simulink model "momentum_dumping"  (R2023b)
settings: Solver=VariableStepAuto  StartTime=0.0  StopTime=30  FixedStep=0.  RelTol=2.8421709430404007E-14
model workspace (MAT data in the model file):
  x0 = 0
values from neighbouring files (symbols this model uses):
  A_BP = A_PB'    [mass_properties.m]
  A_PB = [e1_B'; e2_B'; e3_B']    [mass_properties.m]
  dt_delay = 0.01    [main_momentum.m]
  hwdotmax = 0.004    [main_momentum.m]
  hwmax = 0.015    [main_momentum.m]
  hwstar_B = [0;0;0]    [main_momentum.m]
  J_C_B = Js_C_B + Jd_C_B    [mass_properties.m]
  K = 1/bode(Co*CLTF1*Go,w_crossover_o)    [main_momentum.m]
  Kd = diag([Kd1; Kd2; Kd3])    [main_momentum.m]
  Km = 1/bode(Gm, 2*pi*0.001)    [main_momentum.m]
  Kp = 1/bode(CLTF1/s, 2*pi*0.92244)    [main_momentum.m]
  md = 0.05290847    [mass_properties.m]
  Mmax = 0.17    [main_momentum.m]
  ms = 3.21000120    (= 3.2100012)    [mass_properties.m]
  p = 100*2*pi    (= 628.318530718)    [main_momentum.m]
  q_PB = A2q(A_PB)    [mass_properties.m]
  qstar_BI = e2q(e,150*pi/180)    [main_momentum.m]
  rcb_B = ((ms * rsb_B) + (md * rdb_B)) / (ms + md)    [mass_properties.m]
  rlb_B = [0.16364; -0.03142; -0.02136]    [mass_properties.m]
  s = tf('s')    [main_momentum.m]
  safety = 0.5    [main_momentum.m]
  tau = 1/(100*2*pi)    (= 0.00159154943092)    [main_momentum.m]
  wn = 2*pi*10    (= 62.8318530718)    [main_momentum.m]
  z = 0.006*2*pi    (= 0.0376991118431)    [main_momentum.m]
  zeta = sqrt(2)/2    [main_momentum.m]
undefined symbols (not defined in the file or in its folder): input, input_dis, q0_BI, X, Y, Z
libraries: sm_lib x10, nesl_utility x4, matrix_library x1
settings Model: Creator=bbingham  LastModifiedBy=alanb
settings SolverCC: AlgebraicLoopSolver=TrustRegion
settings DataIOCC: SaveOutput=off  SignalLogging=off  DSMLogging=off  ReturnWorkspaceOutputs=off
settings DebuggingCC: UnconnectedInputMsg=warning  UnconnectedOutputMsg=warning  UnconnectedLineMsg=warning  ArithmeticOperatorsInVariantConditions=warning
settings ModelReferenceCC: EnableRefExpFcnMdlSchedulingChecks=on
settings SFSimCC: SimUseLocalCustomCode=off  CustomCodeUndefinedFunction=UseInterfaceOnly
settings RTWCC: Description=Simulink Desktop Real-Time  SystemTargetFile=sldrt.tlc  TemplateMakefile=sldrt.tmf  RTWUseLocalCustomCode=off  RTWCompilerOptimization=on
settings CodeAppCC: MaxIdLength=95  StateflowObjectComments=on
settings SimulinkDesktopRealTimeCC: TargetPreCompLibLocation=C:\Program Files\MATLAB\R2020a\toolbox\sldrt\lib\win64
settings SimscapeCC: SimscapeNormalizeSystem=off

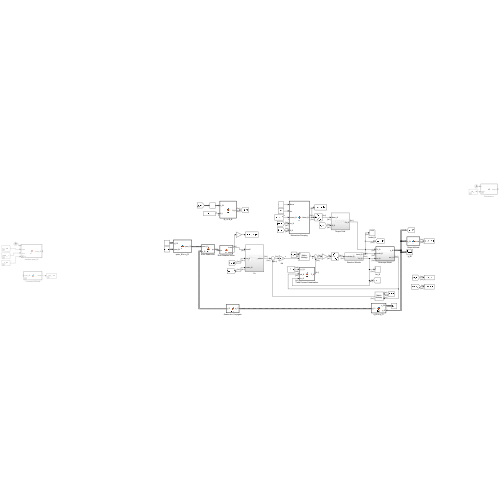
[thumbnail: Simulink's stored preview of the top-level diagram]
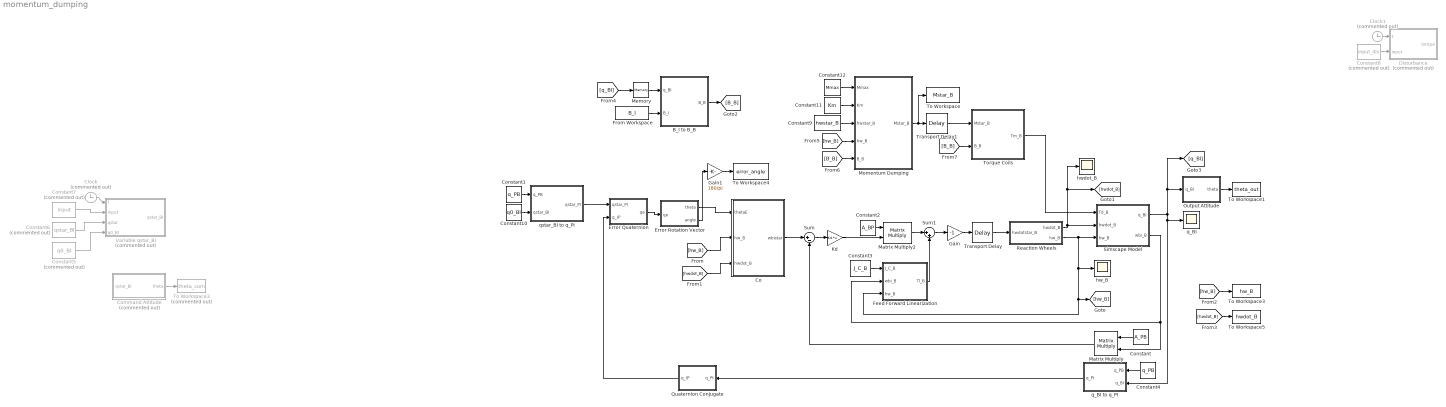
== system momentum_dumping ==
  B_I to B_B : MATLAB Function  TreatAsAtomicUnit=on
  Clock : Clock  Commented=on
  Clock1 : Clock  Commented=on
  Co : Subsystem
  Command Attitude : MATLAB Function  Commented=on  TreatAsAtomicUnit=on
  Constant : Constant  Value=A_PB
  Constant1 : Constant  Value=q_PB  OutDataTypeStr=Bus: qBus
  Constant10 : Constant  Value=q0_BI  OutDataTypeStr=Bus: qBus
  Constant11 : Constant  Value=Km
  Constant12 : Constant  Value=Mmax
  Constant2 : Constant  Value=A_BP
  Constant3 : Constant  Value=J_C_B
  Constant4 : Constant  Value=q_PB  OutDataTypeStr=Bus: qBus
  Constant5 : Constant  Commented=on  Value=q0_BI  OutDataTypeStr=Bus: qBus
  Constant6 : Constant  Commented=on  Value=qstar_BI  OutDataTypeStr=Bus: qBus
  Constant7 : Constant  Commented=on  Value=input
  Constant8 : Constant  Commented=on  Value=input_dis
  Constant9 : Constant  Value=hwstar_B
  Disturbance : MATLAB Function  Commented=on  TreatAsAtomicUnit=on
  Error Quaternion : MATLAB Function  TreatAsAtomicUnit=on
  Error Rotation Vector : MATLAB Function  TreatAsAtomicUnit=on
  Feed Forward Linearization : MATLAB Function  TreatAsAtomicUnit=on
  From Workspace : FromWorkspace  VariableName=B_I
  Gain : Gain  Gain=-1
  Gain1 : Gain  Gain=180/pi
  Kd : Gain  Gain=Kd  Multiplication=Matrix(K*u) (u vector)
  Matrix Multiply : Product  Multiplication=Matrix(*)
  Matrix Multiply2 : Product  Multiplication=Matrix(*)
  Memory : Memory  InitialCondition=q0_BI
  Momentum Dumping : MATLAB Function  TreatAsAtomicUnit=on
  Output Attitude : MATLAB Function  TreatAsAtomicUnit=on
  Quaternion Conjugate : MATLAB Function  TreatAsAtomicUnit=on
  Reaction Wheels : Subsystem
  Simscape Model : Subsystem  TreatAsAtomicUnit=on
  Sum : Sum  Inputs=|+-
  Sum1 : Sum  Inputs=|++
  To Workspace : ToWorkspace  VariableName=Mstar_B  SaveFormat=Timeseries  SampleTime=-1
  To Workspace1 : ToWorkspace  VariableName=theta_out  SaveFormat=Timeseries  SampleTime=-1
  To Workspace2 : ToWorkspace  Commented=on  VariableName=theta_com  SaveFormat=Timeseries  SampleTime=-1
  To Workspace3 : ToWorkspace  VariableName=hw_B  SaveFormat=Timeseries  SampleTime=-1
  To Workspace4 : ToWorkspace  VariableName=error_angle  SaveFormat=Timeseries  SampleTime=-1
  To Workspace5 : ToWorkspace  VariableName=hwdot_B  SaveFormat=Timeseries  SampleTime=-1
  Torque Coils : Subsystem
  Transport Delay : TransportDelay  DelayTime=dt_delay  BufferSize=2048
  Transport Delay1 : TransportDelay  DelayTime=dt_delay  BufferSize=2048
  Variable qstar_BI : MATLAB Function  Commented=on  TreatAsAtomicUnit=on
  hw_B : Scope
  hwdot_B : Scope
  q_BI : Scope
  q_BI to q_PI : MATLAB Function  TreatAsAtomicUnit=on
  qstar_BI to q_PI : MATLAB Function  TreatAsAtomicUnit=on
  wires:
  Simscape Model/2(wbi_B) -> Matrix Multiply/2, Feed Forward Linearization/2(wbi_B)
  Simscape Model/1(q_BI) -> q_BI/1, q_BI to q_PI/2(q_BI), [q_BI], Output Attitude/1(q_BI)
  Constant/1 -> Matrix Multiply/1
  Matrix Multiply/1 -> Sum/2
  Sum/1 -> Kd/1
  Constant2/1 -> Matrix Multiply2/1
  Matrix Multiply2/1 -> Sum1/1
  Feed Forward Linearization/1(Tl_B) -> Sum1/2
  Constant3/1 -> Feed Forward Linearization/1(J_C_B)
  Constant4/1 -> q_BI to q_PI/1(q_PB)
  q_BI to q_PI/1(q_PI) -> Quaternion Conjugate/1(q_PI)
  Quaternion Conjugate/1(q_IP) -> Error Quaternion/2(q_IP)
  Error Quaternion/1(qe) -> Error Rotation Vector/1(qe)
  Clock/1 -> Variable qstar_BI/1(t)
  Error Rotation Vector/1(theta) -> Co/1(thetaE)
  Constant6/1 -> Variable qstar_BI/3(qstar)
  Constant5/1 -> Variable qstar_BI/4(q0_BI)
  Constant7/1 -> Variable qstar_BI/2(input)
  Output Attitude/1(theta) -> To Workspace1/1
  Command Attitude/1(theta) -> To Workspace2/1
  Constant8/1 -> Disturbance/2(input)
  Clock1/1 -> Disturbance/1(t)
  Sum1/1 -> Gain/1
  Gain/1 -> Transport Delay/1
  Transport Delay/1 -> Reaction Wheels/1(hwdotstar_B)
  Reaction Wheels/1(hwdot_B) -> Simscape Model/2(hwdot_B), [hwdot_B], hwdot_B/1
  Reaction Wheels/2(hw_B) -> [hw_B], Feed Forward Linearization/3(hw_B), hw_B/1, Simscape Model/3(hw_B)
  Co/1(wbistar) -> Sum/1
  [hw_B] -> Co/2(hw_B)
  [hwdot_B] -> Co/3(hwdot_B)
  Constant1/1 -> qstar_BI to q_PI/1(q_PB)
  Kd/1 -> Matrix Multiply2/2
  [hw_B] -> To Workspace3/1
  [hwdot_B] -> To Workspace5/1
  qstar_BI to q_PI/1(qstar_PI) -> Error Quaternion/1(qstar_PI)
  Constant10/1 -> qstar_BI to q_PI/2(qstar_BI)
  B_I to B_B/1(B_B) -> [B_B]
  From Workspace/1 -> B_I to B_B/2(B_I)
  [q_BI] -> Memory/1
  Memory/1 -> B_I to B_B/1(q_BI)
  [hw_B] -> Momentum Dumping/4(hw_B)
  [B_B] -> Momentum Dumping/5(B_B)
  Constant9/1 -> Momentum Dumping/3(hwstar_B)
  Constant11/1 -> Momentum Dumping/2(Km)
  Constant12/1 -> Momentum Dumping/1(Mmax)
  Momentum Dumping/1(Mstar_B) -> To Workspace/1, Transport Delay1/1
  Transport Delay1/1 -> Torque Coils/1(Mstar_B)
  [B_B] -> Torque Coils/2(B_B)
  Torque Coils/1(Tm_B) -> Simscape Model/1(Td_B)
  Error Rotation Vector/2(angle) -> Gain1/1
  Gain1/1 -> To Workspace4/1

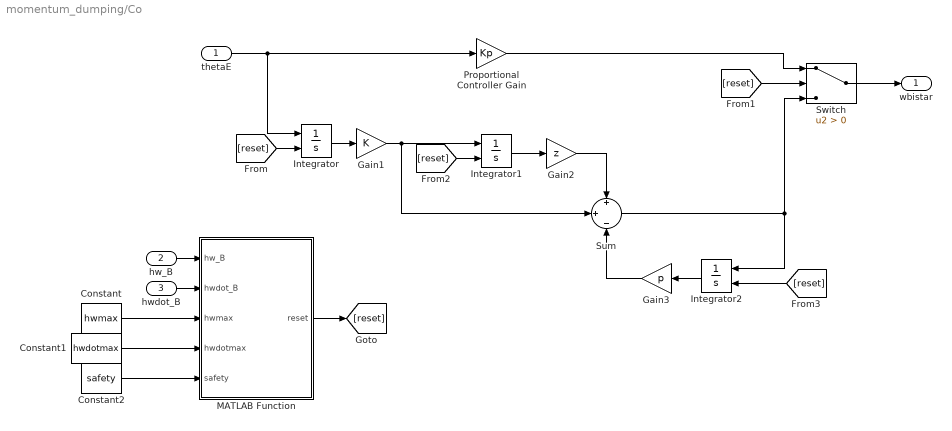
== system momentum_dumping/Co ==
  thetaE : Inport
  hw_B : Inport  Port=2
  hwdot_B : Inport  Port=3
  Constant : Constant  Value=hwmax
  Constant1 : Constant  Value=hwdotmax
  Constant2 : Constant  Value=safety
  Gain1 : Gain  Gain=K
  Gain2 : Gain  Gain=z
  Gain3 : Gain  Gain=p
  Integrator : Integrator  ExternalReset=level
  Integrator1 : Integrator  ExternalReset=level
  Integrator2 : Integrator  ExternalReset=level
  MATLAB Function : MATLAB Function  TreatAsAtomicUnit=on
  Proportional Controller Gain : Gain  Gain=Kp
  Sum : Sum  Inputs=+|+|-
  Switch : Switch  Criteria=u2 > Threshold  SaturateOnIntegerOverflow=off  InputSameDT=off
  wbistar : Outport
  wires:
  thetaE/1 -> Proportional Controller Gain/1, Integrator/1
  hw_B/1 -> MATLAB Function/1(hw_B)
  hwdot_B/1 -> MATLAB Function/2(hwdot_B)
  Constant/1 -> MATLAB Function/3(hwmax)
  Constant1/1 -> MATLAB Function/4(hwdotmax)
  Constant2/1 -> MATLAB Function/5(safety)
  MATLAB Function/1(reset) -> [reset]
  Integrator/1 -> Gain1/1
  Switch/1 -> wbistar/1
  Proportional Controller Gain/1 -> Switch/1
  [reset] -> Switch/2
  [reset] -> Integrator/2
  [reset] -> Integrator1/2
  Gain1/1 -> Sum/2, Integrator1/1
  Integrator1/1 -> Gain2/1
  Gain2/1 -> Sum/1
  Sum/1 -> Integrator2/1, Switch/3
  Integrator2/1 -> Gain3/1
  Gain3/1 -> Sum/3
  [reset] -> Integrator2/2

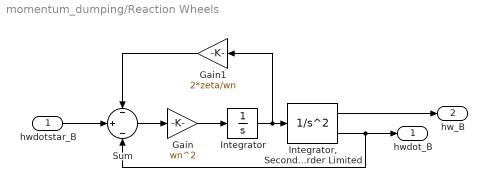
== system momentum_dumping/Reaction Wheels ==
  hwdotstar_B : Inport
  Gain : Gain  Gain=wn^2
  Gain1 : Gain  Gain=2*zeta/wn
  Integrator : Integrator
  "Integrator, Second-Order Limited" : SecondOrderIntegrator  ICX=hw0_B  LimitX=on  UpperLimitX=hwmax  LowerLimitX=-hwmax  LimitDXDT=on  UpperLimitDXDT=hwdotmax  LowerLimitDXDT=-hwdotmax
  Sum : Sum  Inputs=-|+|-
  hwdot_B : Outport
  hw_B : Outport  Port=2
  wires:
  hwdotstar_B/1 -> Sum/2
  Sum/1 -> Gain/1
  Gain1/1 -> Sum/1
  Gain/1 -> Integrator/1
  Integrator/1 -> Gain1/1, "Integrator, Second-Order Limited"/1
  "Integrator, Second-Order Limited"/1 -> hw_B/1
  "Integrator, Second-Order Limited"/2 -> Sum/3, hwdot_B/1

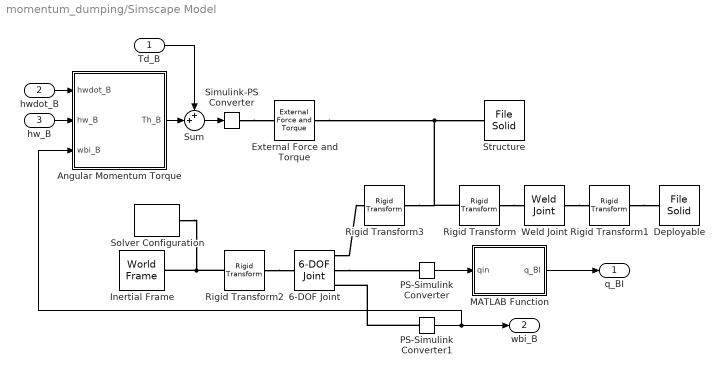
== system momentum_dumping/Simscape Model ==
  Td_B : Inport
  hwdot_B : Inport  Port=2
  hw_B : Inport  Port=3
  6-DOF Joint : sm_lib/Joints/6-DOF Joint  JointMode=Normal  SenseConstraintForce=off  SenseConstraintForceX=off  SenseConstraintForceY=off  SenseConstraintForceZ=off  SenseConstraintTorque=off  SenseConstraintTorqueX=off  SenseConstraintTorqueY=off  SenseConstraintTorqueZ=off  SenseTotalForce=off  SenseTotalForceX=off  SenseTotalForceY=off  SenseTotalForceZ=off  SenseTotalTorque=off  SenseTotalTorqueX=off  SenseTotalTorqueY=off  SenseTotalTorqueZ=off  CompositeWrenchDir=FollowerOnBase  CompositeWrenchFrame=BaseFrame  PxEquilibriumPosition=0  PxEquilibriumPositionUnits=m  PxSpringStiffness=0  PxSpringStiffnessUnits=N/m  PxDampingCoefficient=0  PxDampingCoefficientUnits=N/(m/s)  PxTorqueActuationMode=NoTorque  PxMotionActuationMode=ComputedMotion  PxSensePosition=off  PxSenseVelocity=off  PxSenseAcceleration=off  PxSenseTorqueForce=off  PxSenseLowerLimitTorqueForce=off  PxSenseUpperLimitTorqueForce=off  PxLowerLimitSpecify=off  PxLowerLimitBound=-1  PxLowerLimitBoundUnits=m  PxLowerLimitStiffness=1e6  PxLowerLimitStiffnessUnits=N/m  PxLowerLimitDamping=1e3  PxLowerLimitDampingUnits=N/(m/s)  PxLowerLimitTransitionRegionWidth=1e-4  PxLowerLimitTransitionRegionWidthUnits=m  PxUpperLimitSpecify=off  PxUpperLimitBound=1  PxUpperLimitBoundUnits=m  PxUpperLimitStiffness=1e6  PxUpperLimitStiffnessUnits=N/m  PxUpperLimitDamping=1e3  PxUpperLimitDampingUnits=N/(m/s)  PxUpperLimitTransitionRegionWidth=1e-4  PxUpperLimitTransitionRegionWidthUnits=m  PxPositionTargetSpecify=off  PxPositionTargetPriority=High  PxPositionTargetValue=0  PxPositionTargetValueUnits=m  PxVelocityTargetSpecify=off  PxVelocityTargetPriority=High  PxVelocityTargetValue=0  PxVelocityTargetValueUnits=m/s  PyEquilibriumPosition=0  PyEquilibriumPositionUnits=m  PySpringStiffness=0  PySpringStiffnessUnits=N/m  PyDampingCoefficient=0  PyDampingCoefficientUnits=N/(m/s)  PyTorqueActuationMode=NoTorque  PyMotionActuationMode=ComputedMotion  PySensePosition=off  PySenseVelocity=off  PySenseAcceleration=off  PySenseTorqueForce=off  PySenseLowerLimitTorqueForce=off  PySenseUpperLimitTorqueForce=off  PyLowerLimitSpecify=off  PyLowerLimitBound=-1  PyLowerLimitBoundUnits=m  PyLowerLimitStiffness=1e6  PyLowerLimitStiffnessUnits=N/m  PyLowerLimitDamping=1e3  PyLowerLimitDampingUnits=N/(m/s)  PyLowerLimitTransitionRegionWidth=1e-4  PyLowerLimitTransitionRegionWidthUnits=m  PyUpperLimitSpecify=off  PyUpperLimitBound=1  PyUpperLimitBoundUnits=m  PyUpperLimitStiffness=1e6  PyUpperLimitStiffnessUnits=N/m  PyUpperLimitDamping=1e3  PyUpperLimitDampingUnits=N/(m/s)  PyUpperLimitTransitionRegionWidth=1e-4  PyUpperLimitTransitionRegionWidthUnits=m  PyPositionTargetSpecify=off  PyPositionTargetPriority=High  PyPositionTargetValue=0  PyPositionTargetValueUnits=m  PyVelocityTargetSpecify=off  PyVelocityTargetPriority=High  PyVelocityTargetValue=0  PyVelocityTargetValueUnits=m/s  PzEquilibriumPosition=0  PzEquilibriumPositionUnits=m  PzSpringStiffness=0  PzSpringStiffnessUnits=N/m  PzDampingCoefficient=0  PzDampingCoefficientUnits=N/(m/s)  PzTorqueActuationMode=NoTorque  PzMotionActuationMode=ComputedMotion  PzSensePosition=off  PzSenseVelocity=off  PzSenseAcceleration=off  PzSenseTorqueForce=off  PzSenseLowerLimitTorqueForce=off  PzSenseUpperLimitTorqueForce=off  PzLowerLimitSpecify=off  PzLowerLimitBound=-1  PzLowerLimitBoundUnits=m  PzLowerLimitStiffness=1e6  PzLowerLimitStiffnessUnits=N/m  PzLowerLimitDamping=1e3  PzLowerLimitDampingUnits=N/(m/s)  PzLowerLimitTransitionRegionWidth=1e-4  PzLowerLimitTransitionRegionWidthUnits=m  PzUpperLimitSpecify=off  PzUpperLimitBound=1  PzUpperLimitBoundUnits=m  PzUpperLimitStiffness=1e6  PzUpperLimitStiffnessUnits=N/m  PzUpperLimitDamping=1e3  PzUpperLimitDampingUnits=N/(m/s)  PzUpperLimitTransitionRegionWidth=1e-4  PzUpperLimitTransitionRegionWidthUnits=m  PzPositionTargetSpecify=off  PzPositionTargetPriority=High  PzPositionTargetValue=0  PzPositionTargetValueUnits=m  PzVelocityTargetSpecify=off  PzVelocityTargetPriority=High  PzVelocityTargetValue=0  PzVelocityTargetValueUnits=m/s  SphEqPosRotationMethod=None  SphEqPosRotationAngleUnits=deg  SphEqPosRotationStandardAxis=+Z  SphEqPosRotationAngle=0.0  SphEqPosRotationArbitraryAxis=[0 0 1]  SphEqPosFollAlignAxisA=+X  SphEqPosBaseAlignAxisA=+Y  SphEqPosFollAlignAxisB=+Y  SphEqPosBaseAlignAxisB=+Z  SphEqPosRotationSequenceAxes=FollowerAxes  SphEqPosRotationSequence=XYX  SphEqPosRotationSequenceAngles=[0 0 0]  SphEqPosRotationSequenceAnglesUnits=deg  SphEqPosRotationMatrix=[1 0 0; 0 1 0; 0 0 1]  SphEqPosQuaternion=[1 0 0 0]  SphSpringStiffness=0  SphSpringStiffnessUnits=N*m/deg  SphDampingCoefficient=0  SphDampingCoefficientUnits=N*m/(deg/s)  SphActuateTorqueX=off  SphActuateTorqueY=off  SphActuateTorqueZ=off  SphActuateTorque=off  SphTorqueActuationMode=NoTorque  SphMotionActuationMode=ComputedMotion  SphActuationFrame=BaseFrame  SphSensePosition=on  SphSenseVelocityX=off  SphSenseVelocityY=off  SphSenseVelocityZ=off  SphSenseVelocity=on  SphSenseAccelerationX=off  SphSenseAccelerationY=off  SphSenseAccelerationZ=off  SphSenseAcceleration=off  SphSenseTorqueX=off  SphSenseTorqueY=off  SphSenseTorqueZ=off  SphSenseTorqueForce=off  SphSenseLowerLimitTorqueMag=off  SphSenseUpperLimitTorqueMag=off  SphSensingFrame=FollowerFrame  SphLowerLimitSpecify=off  SphLowerLimitBound=15  SphLowerLimitBoundUnits=deg  SphLowerLimitStiffness=1e4  SphLowerLimitStiffnessUnits=N*m/deg  SphLowerLimitDamping=10  SphLowerLimitDampingUnits=N*m/(deg/s)  SphLowerLimitTransitionRegionWidth=0.1  SphLowerLimitTransitionRegionWidthUnits=deg  SphUpperLimitSpecify=off  SphUpperLimitBound=45  SphUpperLimitBoundUnits=deg  SphUpperLimitStiffness=1e4  SphUpperLimitStiffnessUnits=N*m/deg  SphUpperLimitDamping=10  SphUpperLimitDampingUnits=N*m/(deg/s)  SphUpperLimitTransitionRegionWidth=0.1  SphUpperLimitTransitionRegionWidthUnits=deg  SphPositionTargetRotationMethod=RotationMatrix  SphPositionTargetRotationAngleUnits=deg  SphPositionTargetRotationStandardAxis=+Z  SphPositionTargetRotationAngle=0.0  SphPositionTargetRotationArbitraryAxis=[0 0 1]  SphPositionTargetFollAlignAxisA=+X  SphPositionTargetBaseAlignAxisA=+Y  SphPositionTargetFollAlignAxisB=+Y  SphPositionTargetBaseAlignAxisB=+Z  SphPositionTargetRotationSequenceAxes=FollowerAxes  SphPositionTargetRotationSequence=XYX  SphPositionTargetRotationSequenceAngles=[0 0 0]  SphPositionTargetRotationSequenceAnglesUnits=deg  SphPositionTargetRotationMatrix=A0_IB  SphPositionTargetQuaternion=[1 0 0 0]  SphPositionTargetSpecify=on  SphPositionTargetPriority=High  SphVelocityTargetValue=wbi0_B  SphVelocityTargetValueUnits=rad/s  SphVelocityTargetSpecify=on  SphVelocityTargetPriority=High  SphVelocityTargetInFollowerFrame=on
  Angular Momentum Torque : MATLAB Function  TreatAsAtomicUnit=on
  Deployable : sm_lib/Body Elements/File Solid  ExtGeomFileName=C:\Users\alanb\OneDrive\Documents\Homework Spring 2024\Spacecraft Attitude Control Theory\03 Attitude Dynamics\Deployable.STL  UnitType=Custom  ExtGeomFileUnits=mm  StepReaderType=HEX  ExportConvexHullGeometry=off  InertiaType=Custom  Mass=md  MassUnits=kg  CenterOfMass=rdb_B  CenterOfMassUnits=m  MomentsOfInertia=Md_D_B  MomentsOfInertiaUnits=kg*m^2  ProductsOfInertia=Pd_D_B  ProductsOfInertiaUnits=kg*m^2  BasedOnType=DensityFromFile  Density=1000  DensityUnits=kg/m^3  DoExposeReferenceFrame=on  SerializedFrames=<Frames/>  GraphicType=FromGeometry  MarkerShape=Sphere  MarkerSize=10  GraphicVisPropType=SimpleVisualProperties  GraphicDiffuseColor=[0.2 0.6 1.0]  GraphicSpecularColor=[0.5 0.5 0.5 1.0]  GraphicAmbientColor=[0.15 0.15 0.15 1.0]  GraphicEmissiveColor=[0.0 0.0 0.0 1.0]  GraphicShininess=75  GraphicOpacity=1.0
  External Force and Torque : sm_lib/Forces and Torques/External Force and Torque  ForceResolutionFrame=AttachedFrame  EnableForceX=off  EnableForceY=off  EnableForceZ=off  EnableForce=off  TorqueResolutionFrame=AttachedFrame  EnableTorqueX=off  EnableTorqueY=off  EnableTorqueZ=off  EnableTorque=on
  Inertial Frame : sm_lib/Frames and Transforms/World Frame
  MATLAB Function : MATLAB Function  TreatAsAtomicUnit=on
  PS-Simulink Converter : nesl_utility/PS-Simulink Converter  PhysicalDomain=network_engine_domain  SubClassName=ps_output  LeftPortType=input  RightPortType=output  PseudoPeriodic=off  Frequencies=[]  VectorFormat=inherit  Unit=inherit  AffineConversion=off
  PS-Simulink Converter1 : nesl_utility/PS-Simulink Converter  PhysicalDomain=network_engine_domain  SubClassName=ps_output  LeftPortType=input  RightPortType=output  PseudoPeriodic=off  Frequencies=[]  VectorFormat=inherit  Unit=inherit  AffineConversion=off
  Rigid Transform : sm_lib/Frames and Transforms/Rigid Transform  TranslationMethod=Cartesian  TranslationStandardOffset=0  TranslationStandardOffsetUnits=m  TranslationStandardAxis=+Z  TranslationCartesianOffset=rlb_B  TranslationCartesianOffsetUnits=m  TranslationROffset=0  TranslationROffsetUnits=m  TranslationZOffset=0  TranslationZOffsetUnits=m  TranslationThetaOffset=0  TranslationThetaOffsetUnits=deg  RotationMethod=None  RotationAngleUnits=deg  RotationStandardAxis=+Z  RotationAngle=0.0  RotationArbitraryAxis=[0 0 1]  FollAlignAxisA=+X  BaseAlignAxisA=+Y  FollAlignAxisB=+Y  BaseAlignAxisB=+Z  RotationSequenceAxes=FollowerAxes  RotationSequence=XYX  RotationSequenceAngles=[0 0 0]  RotationSequenceAnglesUnits=deg  RotationMatrix=[1 0 0; 0 1 0; 0 0 1]  Quaternion=[1 0 0 0]
  Rigid Transform1 : sm_lib/Frames and Transforms/Rigid Transform  TranslationMethod=Cartesian  TranslationStandardOffset=0  TranslationStandardOffsetUnits=m  TranslationStandardAxis=+Z  TranslationCartesianOffset=-rlb_B  TranslationCartesianOffsetUnits=m  TranslationROffset=0  TranslationROffsetUnits=m  TranslationZOffset=0  TranslationZOffsetUnits=m  TranslationThetaOffset=0  TranslationThetaOffsetUnits=deg  RotationMethod=None  RotationAngleUnits=deg  RotationStandardAxis=+Z  RotationAngle=0.0  RotationArbitraryAxis=[0 0 1]  FollAlignAxisA=+X  BaseAlignAxisA=+Y  FollAlignAxisB=+Y  BaseAlignAxisB=+Z  RotationSequenceAxes=FollowerAxes  RotationSequence=XYX  RotationSequenceAngles=[0 0 0]  RotationSequenceAnglesUnits=deg  RotationMatrix=[1 0 0; 0 1 0; 0 0 1]  Quaternion=[1 0 0 0]
  Rigid Transform2 : sm_lib/Frames and Transforms/Rigid Transform  TranslationMethod=Cartesian  TranslationStandardOffset=0  TranslationStandardOffsetUnits=m  TranslationStandardAxis=+Z  TranslationCartesianOffset=rcb_B  TranslationCartesianOffsetUnits=m  TranslationROffset=0  TranslationROffsetUnits=m  TranslationZOffset=0  TranslationZOffsetUnits=m  TranslationThetaOffset=0  TranslationThetaOffsetUnits=deg  RotationMethod=None  RotationAngleUnits=deg  RotationStandardAxis=+Z  RotationAngle=0.0  RotationArbitraryAxis=[0 0 1]  FollAlignAxisA=+X  BaseAlignAxisA=+Y  FollAlignAxisB=+Y  BaseAlignAxisB=+Z  RotationSequenceAxes=FollowerAxes  RotationSequence=XYX  RotationSequenceAngles=[0 0 0]  RotationSequenceAnglesUnits=deg  RotationMatrix=[1 0 0; 0 1 0; 0 0 1]  Quaternion=[1 0 0 0]
  Rigid Transform3 : sm_lib/Frames and Transforms/Rigid Transform  TranslationMethod=Cartesian  TranslationStandardOffset=0  TranslationStandardOffsetUnits=m  TranslationStandardAxis=+Z  TranslationCartesianOffset=-rcb_B  TranslationCartesianOffsetUnits=m  TranslationROffset=0  TranslationROffsetUnits=m  TranslationZOffset=0  TranslationZOffsetUnits=m  TranslationThetaOffset=0  TranslationThetaOffsetUnits=deg  RotationMethod=None  RotationAngleUnits=deg  RotationStandardAxis=+Z  RotationAngle=0.0  RotationArbitraryAxis=[0 0 1]  FollAlignAxisA=+X  BaseAlignAxisA=+Y  FollAlignAxisB=+Y  BaseAlignAxisB=+Z  RotationSequenceAxes=FollowerAxes  RotationSequence=XYX  RotationSequenceAngles=[0 0 0]  RotationSequenceAnglesUnits=deg  RotationMatrix=[1 0 0; 0 1 0; 0 0 1]  Quaternion=[1 0 0 0]
  Simulink-PS Converter : nesl_utility/Simulink-PS Converter  PhysicalDomain=network_engine_domain  SubClassName=ps_input  LeftPortType=input  RightPortType=output  PseudoPeriodic=off  Frequencies=[]  NoiseDistribution=none  NoiseParameters=[]  Unit=1  AffineConversion=off  FilteringAndDerivatives=provide  SimscapeFilterOrder=1  InputFilterTimeConstant=0.001  UdotUserProvided=0
  Solver Configuration : nesl_utility/Solver Configuration  PhysicalDomain=network_engine_domain  SubClassName=solver  LeftPortType=input  RightPortType=generic  Tones=[]  Harmonics=[]  SimulateNoise=off  Profile=off  UseLocalSampling=off  EnableSwitchedLinearOptims=on  FrequencyDomain=off  UseCCode=off  RelTol=0.001  AbsTol=0.001  MinStep=1e-09  ToWorkspace=off  RevertToSquareIcSolve=off  NumHomotopyIterations=100  PhasorMode=off  PhasorModeNumHarmonics=1  ConsistencySolver=NEWTON_XTOL_AFTER_FTOL  IndexReductionMethod=DerivativeReplacement  DoDC=off  ResidualTolerance=1e-09  ConsistencyTolSource=GLOBAL  ConsistencyAbsTol=0.001  ConsistencyRelTol=0.001  ConsistencyTolFactor=1  UseLocalSolver=off  LocalSolverChoice=NE_BACKWARD_EULER_ADVANCER  ResolveIndetEquations=on  FunctionEvalNumThread=1  LocalSolverSampleTime=0.001  DoFixedCost=off  MaxNonlinIter=3  MaxModeIter=2  ComputeImpulses=off  ImpulseIterations=2  LinearAlgebra=auto  LinearAlgebraNumThread=0  EquationFormulation=NE_TIME_EF  DelaysMemoryBudget=1024  AutomaticFiltering=on  FilteringTimeConstant=0.001  PartitionStorageMethod=AS_NEEDED  PartitionMemoryBudget=1024  PartitionMethod=ROBUST  MultibodyUseLocalSolver=off  MultibodyLocalSolverChoice=ODE1  MultibodyLocalSolverSampleTime=0.001
  Structure : sm_lib/Body Elements/File Solid  ExtGeomFileName=C:\Users\alanb\OneDrive\Documents\Homework Spring 2024\Spacecraft Attitude Control Theory\03 Attitude Dynamics\Structure.STL  UnitType=Custom  ExtGeomFileUnits=mm  StepReaderType=HEX  ExportConvexHullGeometry=off  InertiaType=Custom  Mass=ms  MassUnits=kg  CenterOfMass=rsb_B  CenterOfMassUnits=m  MomentsOfInertia=Ms_S_B  MomentsOfInertiaUnits=kg*m^2  ProductsOfInertia=Ps_S_B  ProductsOfInertiaUnits=kg*m^2  BasedOnType=DensityFromFile  Density=1000  DensityUnits=kg/m^3  DoExposeReferenceFrame=on  SerializedFrames=<Frames/>  GraphicType=FromGeometry  MarkerShape=Sphere  MarkerSize=10  GraphicVisPropType=SimpleVisualProperties  GraphicDiffuseColor=[1.0 0.4 0.4]  GraphicSpecularColor=[0.5 0.5 0.5 1.0]  GraphicAmbientColor=[0.15 0.15 0.15 1.0]  GraphicEmissiveColor=[0.0 0.0 0.0 1.0]  GraphicShininess=75  GraphicOpacity=1.0
  Sum : Sum  Inputs=++|
  Weld Joint : sm_lib/Joints/Weld Joint  JointMode=Normal  SenseConstraintForce=off  SenseConstraintForceX=off  SenseConstraintForceY=off  SenseConstraintForceZ=off  SenseConstraintTorque=off  SenseConstraintTorqueX=off  SenseConstraintTorqueY=off  SenseConstraintTorqueZ=off  SenseTotalForce=off  SenseTotalForceX=off  SenseTotalForceY=off  SenseTotalForceZ=off  SenseTotalTorque=off  SenseTotalTorqueX=off  SenseTotalTorqueY=off  SenseTotalTorqueZ=off  CompositeWrenchDir=FollowerOnBase  CompositeWrenchFrame=BaseFrame
  q_BI : Outport  OutDataTypeStr=Bus: qBus  VectorParamsAs1DForOutWhenUnconnected=off
  wbi_B : Outport  Port=2  VectorParamsAs1DForOutWhenUnconnected=off
  wires:
  PS-Simulink Converter/1 -> MATLAB Function/1(qin)
  MATLAB Function/1(q_BI) -> q_BI/1
  PS-Simulink Converter1/1 -> Angular Momentum Torque/3(wbi_B), wbi_B/1
  Sum/1 -> Simulink-PS Converter/1
  Td_B/1 -> Sum/1
  Angular Momentum Torque/1(Th_B) -> Sum/2
  hwdot_B/1 -> Angular Momentum Torque/1(hwdot_B)
  hw_B/1 -> Angular Momentum Torque/2(hw_B)
  connections:
  Solver Configuration/RConn1 -- Inertial Frame/RConn1 -- Rigid Transform2/LConn1
  External Force and Torque/RConn1 -- Rigid Transform3/RConn1 -- Rigid Transform/LConn1 -- Structure/RConn1
  Simulink-PS Converter/RConn1 -- External Force and Torque/LConn1
  Rigid Transform/RConn1 -- Weld Joint/LConn1
  Weld Joint/RConn1 -- Rigid Transform1/LConn1
  Rigid Transform1/RConn1 -- Deployable/RConn1
  6-DOF Joint/RConn2 -- PS-Simulink Converter/LConn1
  PS-Simulink Converter1/LConn1 -- 6-DOF Joint/RConn3
  Rigid Transform2/RConn1 -- 6-DOF Joint/LConn1
  6-DOF Joint/RConn1 -- Rigid Transform3/LConn1

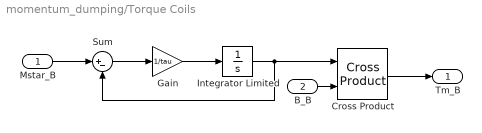
== system momentum_dumping/Torque Coils ==
  Mstar_B : Inport
  B_B : Inport  Port=2
  Cross Product : matrix_library/Cross Product
  Gain : Gain  Gain=1/tau
  Integrator Limited : Integrator  LimitOutput=on  UpperSaturationLimit=Mmax  LowerSaturationLimit=-Mmax  ZeroCross=off
  Sum : Sum  Inputs=|+-
  Tm_B : Outport
  wires:
  Mstar_B/1 -> Sum/1
  Sum/1 -> Gain/1
  Gain/1 -> Integrator Limited/1
  B_B/1 -> Cross Product/2
  Integrator Limited/1 -> Cross Product/1, Sum/2
  Cross Product/1 -> Tm_B/1

== matlab function momentum_dumping/Co/MATLAB Function ==
  data: hw_B input; reset output; hwdot_B input; hwmax input; hwdotmax input; safety input
function reset = fcn(hw_B,hwdot_B,hwmax,hwdotmax,safety)

reset = 0;

if max(abs(hw_B)) >= hwmax*safety || max(abs(hwdot_B)) >= hwdotmax*safety

    reset = 1;

end

== matlab function momentum_dumping/Simscape Model/MATLAB Function ==
  data: qin input; q_BI output Bus: qBus
function q_BI = fcn(qin)

q_BI.s = qin(1);
q_BI.v = qin(2:4);

== matlab function momentum_dumping/B_I to B_B ==
  data: q_BI input Bus: qBus; B_B output; B_I input
function B_B = fcn(q_BI, B_I)

A_BI = q2A(q_BI);

B_B = A_BI*B_I;

== matlab function momentum_dumping/Momentum Dumping ==
  data: Mmax input; Mstar_B output; Km input; hwstar_B input; hw_B input; B_B input
function Mstar_B = fcn(Mmax, Km, hwstar_B, hw_B, B_B)

dh_B = hw_B - hwstar_B;

Mstar_B = -Km/norm(B_B)^2*cross(B_B,dh_B);

Mbig = max(abs(Mstar_B));

if Mbig > Mmax
    Mstar_B = Mstar_B/Mbig*Mmax;
end

== matlab function momentum_dumping/Feed Forward Linearization ==
  data: J_C_B input; Tl_B output; wbi_B input; hw_B input
function Tl_B = fcn(J_C_B, wbi_B, hw_B)

Tl_B = cross(wbi_B, J_C_B*wbi_B + hw_B);

== matlab function momentum_dumping/q_BI to q_PI ==
  data: q_PB input Bus: qBus; q_PI output Bus: qBus; q_BI input Bus: qBus
function q_PI = fcn(q_PB,q_BI)

q_PI = qX(q_PB,q_BI);

== matlab function momentum_dumping/Quaternion Conjugate ==
  data: q_PI input Bus: qBus; q_IP output Bus: qBus
function q_IP = fcn(q_PI)

q_IP = qT(q_PI);

== matlab function momentum_dumping/Error Quaternion ==
  data: qstar_PI input Bus: qBus; qe output Bus: qBus; q_IP input Bus: qBus
function qe = fcn(qstar_PI, q_IP)

qe = qX(qstar_PI,q_IP);

== matlab function momentum_dumping/Error Rotation Vector ==
  data: qe input Bus: qBus; theta output; angle output
function [theta, angle] = fcn(qe)

qe = qUnit(qe);

[e, angle] = q2e(qe);

theta = e*angle;

== matlab function momentum_dumping/qstar_BI to q_PI ==
  data: q_PB input Bus: qBus; qstar_PI output Bus: qBus; qstar_BI input Bus: qBus
function qstar_PI = fcn(q_PB,qstar_BI)

qstar_PI = qX(q_PB,qstar_BI);

== matlab function momentum_dumping/Variable qstar_BI ==
  data: t input; qstar_BI output Bus: qBus; input input; qstar input Bus: qBus; q0_BI input Bus: qBus
function qstar_BI = fcn(t,input,qstar,q0_BI)

e = [1;1;1];

% Command to hold current attitude (set qstar = q0_BI)
if input == 0
    qstar_BI = q0_BI;

% Step command input (set qstar = qstar_BI)
elseif input == 1
    qstar_BI = qstar;

% Ramp command input
elseif input == 2
    qstar_BI = e2q(e, (20*t + 15)*pi/180);

% Sine wave command input
elseif input == 3
    qstar_BI = e2q(e, 5*pi/180 * sin(1.693*2*pi*t));

% Hold current attitude if there is no command
else
    qstar_BI = q0_BI;
end

== matlab function momentum_dumping/Output Attitude ==
  data: q_BI input Bus: qBus; theta output
function theta = fcn(q_BI)

q_BI = qUnit(q_BI);

[e, angle] = q2e(q_BI);

theta = e*angle;

== matlab function momentum_dumping/Command Attitude ==
  data: qstar_BI input Bus: qBus; theta output
function theta = fcn(qstar_BI)

qstar_BI = qUnit(qstar_BI);

[e, angle] = q2e(qstar_BI);

theta = e*angle;

== matlab function momentum_dumping/Disturbance ==
  data: t input; input input; torque output
function torque = fcn(t,input)

% Constant disturbance torque
if input == 1
    torque = [0.001;0.001;0.001];

% Sine wave disturbance torque
elseif input == 2
    torque = [1;1;1] * (5*pi/180 * sin(1.693*2*pi*t));

% No disturbance torque
else
    torque = [0;0;0];
end

== matlab function momentum_dumping/Simscape Model/Angular Momentum Torque ==
  data: hwdot_B input; Th_B output; hw_B input; wbi_B input
function Th_B = fcn(hwdot_B, hw_B, wbi_B)

Th_B = -hwdot_B - cross(wbi_B,hw_B);
